simulink model "app_webserver_demo"  (Simulink 7.3)
settings: Solver=FixedStepDiscrete  SolverMode=SingleTasking  StartTime=0.0  StopTime=10.0  RelTol=1e-3
PreLoadFcn:
  | waijung.modelPreload; % Required for working with Waijung Blockset. Do not remove.
undefined symbols (not defined in the file): A0, A1, A2, A3, A7, B0, B1, B10, B11, B12, B13, C1, C2, C3, C4, C5, HSEOSC, LQFP176, STM32F417IG
libraries: waijung_webserver x3, stm32f4_boot_lib x1, simulink x1, stm32f4_io_lib x1, stm32f4_device_config_lib x1
CloseFcn:
  | waijung.modelClose; % Required for working with Waijung Blockset. Do not remove.
settings Model: Creator=Krisada  LastModifiedBy=Krisada
settings OptimizationCC: OptimizeModelRefInitCode=on  LifeSpan=1
settings HardwareCC: ProdEndianess=LittleEndian  ProdHWDeviceType=ARM Compatible->Cortex - M4  TargetEndianess=LittleEndian  TargetHWDeviceType=ARM Compatible->Cortex - M4
settings RTWCC: SystemTargetFile=stm32f4.tlc  GenerateMakefile=off  TemplateMakefile=ert_default_tmf  Description=STM32F4 Target  ProcessScript=stm32f4_make_rtw_hook
settings CodeAppCC: IgnoreCustomStorageClasses=off
settings STFCustomTargetCC: ModelReferenceCompliant=off  CombineOutputUpdateFcns=on  ERTCustomFileBanners=on  SupportContinuousTime=off  SupportNonInlinedSFcns=off  SystemTargetFile=stm32f4.tlc
settings ERTTargetCC: MultiwordLength=2048  ModelReferenceCompliant=off  ParMdlRefBuildCompliant=off  CompOptLevelCompliant=off  ERTFirstTimeCompliant=off  ModelStepFunctionPrototypeControlCompliant=off  CPPClassGenCompliant=off  ExtModeMexFile=noextcomm  InlinedParameterPlacement=NonHierarchical  ERTSrcFileBannerTemplate=stm32f4_code_template.cgt  ERTHdrFileBannerTemplate=stm32f4_code_template.cgt  ERTDataSrcFileTemplate=stm32f4_code_template.cgt  ERTDataHdrFileTemplate=stm32f4_code_template.cgt  ERTCustomFileTemplate=stm32f4_file_process.tlc

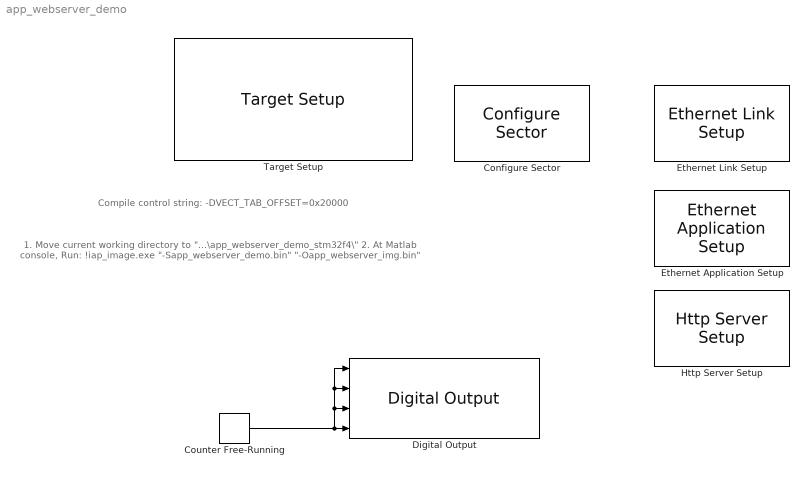
== system app_webserver_demo ==
  note: 1. Move current working directory to "...\app_webserver_demo_stm32f4\"
      | 2. At Matlab console, Run:
      | !iap_image.exe "-Sapp_webserver_demo.bin" "-Oapp_webserver_img.bin"
  note: Compile control string:
      |  -DVECT_TAB_OFFSET=0x20000
  Configure Sector : stm32f4_boot_lib/Configure Sector  conf=Configure  flashorigin=0x8020000  flashlength=0x060000  enableisr=off  usersector=Sector 5: 0x08020000 - 0x0803FFFF  sampletime=-1  sampletimestr=0.001  blockid=ConfigureSector  inputarray=[]  inputlabelarray={}  outputarray=[]  outputlabelarray={}  compat=0  confstr="[\"08020000\",\"5\"]"
  Counter Free-Running : simulink/Sources/Counter Free-Running  SystemSampleTime=-1  NumBits=16  tsamp=0.5
  Digital Output : stm32f4_io_lib/Digital Output  use_bitband=on  port=D  speed=100  porttype=Push Pull  porttypestr=PP  use_pin0=off  use_pin1=off  use_pin2=off  use_pin3=off  use_pin4=off  use_pin5=off  use_pin6=off  use_pin7=off  use_pin8=off  use_pin9=off  use_pin10=off  use_pin11=off  use_pin12=on  use_pin13=on  use_pin14=on  use_pin15=on  pinstr=GPIO_Pin_12 | GPIO_Pin_13 | GPIO_Pin_14 | GPIO_Pin_15  usedpinarray="[0  0  0  0  0  0  0  0  0  0  0  0  1  1  1  1]"  bitbandingstr=|  sampletime=-1  sampletimestr=0.5  blockid=DigitalOutput  enablecustomportlabel=off  globalinit=off  cinputportlabel=In1, In2  coutputportlabel=0
      | #define DigitalOutput_D12 Peripheral_BB(GPIOD->ODR, 12)  /* Output pin */
      | #define DigitalOutput_D13 Peripheral_BB(GPIOD->ODR, 13)  /* Output pin */
      | #define DigitalOutput_D14 Peripheral_BB(GPIOD->ODR, 14)  /* Output pin */
      | #define DigitalOutput_D15 Peripheral_BB(GPIOD->ODR, 15)  /* Output pin */
  Ethernet Application Setup : waijung_webserver/Ethernet Application Setup  conf=Setup  ipaddress=192.168.1.31  netmask=255.255.255.0  gateway=192.168.1.1  macaddress=02-00-00-00-00-00  dhcp=off  timerscaler=10  portpinstr=0  sampletime=0.001  blockid=EthernetApplicationSetup  inputporttype=[]  inputportwidth=[]  inputportlabel={}  outputporttype=[]  outputportwidth=[]  outputportlabel={}  compat=0  optionstring="[\"Dummy\",\"192\",\"168\",\"1\",\"31\",\"255\",\"255\",\"255\",\"0\",\"192\",\"168\",\"1\",\"1\",\"02\",\"00\",\"00\",\"00\",\"00\",\"00\",\"off\",\"10\"]"
  Ethernet Link Setup : waijung_webserver/Ethernet Link Setup  conf=Setup  interfacepin=Profile #1  wj_interfacetype=MII  pin_mdio=A2  pin_mdc=C1  pin_pps=Not used  pin_crs=A0  pin_col=A3  pin_dv=A7  pin_rxclk=A1  pin_rxer=B10  pin_rxd0=C4  pin_rxd1=C5  pin_rxd2=B0  pin_rxd3=B1  pin_txclk=C3  pin_txen=B11  pin_txd0=B12  pin_txd1=B13  pin_txd2=C2  pin_txd3=E2  portpinstr=A0,A1,A2,A3,A7,B0,B1,E2,B10,B11,B12,B13,C1,C2,C3,C4,C5  sampletime=inf  blockid=EthernetLinkSetup  inputporttype=[]  inputportwidth=[]  inputportlabel={}  outputporttype=[]  outputportwidth=[]  outputportlabel={}  compat=0  optionstring="[\"xxx\",\"on\",\"on\",\"on\",\"off\",\"on\",\"off\",\"off\",\"off\",\"off\",\"on\",\"on\",\"on\",\"on\",\"on\",\"on\",\"on\",\"off\",\"on\",\"on\",\"on\",\"on\",\"on\",\"on\",\"on\",\"on\",\"on\",\"on\",\"A\",\"0\",\"A\",\"1\",\"A\",\"2\",\"A\",\"3\",\"A\",\"7\",\"B\",\"0\",\"B\",\"1\",\"N\",\"ot used\",\"E\",\"2\",\"B\",\"10\",\"B\",\"11\",\"B\",\"12\",\"B\",\"13\",\"C\",\"1\",\"C\",\"2\",\"C\",\"3\",\"C\",\"4\",\"C\",\"5\",\"MII\"]"
  Http Server Setup : waijung_webserver/Http Server Setup  conf=Setup  port=80  ssl=Disable  sqlite=Disable  iap=Disable  mempool=8  debugport=Disable  portpinstr=0  sampletime=inf  blockid=HttpServerSetup  inputporttype=[]  inputportwidth=[]  inputportlabel={}  outputporttype=[]  outputportwidth=[]  outputportlabel={}  compat=0  optionstring="[\"80\",\"0\",\"0\",\"Disable\",\"Disable\",\"8\",\"14.03a\",\"\",\"\",\"\"]"
  Target Setup : stm32f4_device_config_lib/Target Setup  Priority=100  compiler=GNU ARM  previous_compiler=GNU ARM  mcu=STM32F417IG (LQFP176)  mcustr=STM32F417IG  clockconfig=HSEOSC-8MHz  system_stm32f4xx_c_path=F:\trunk\targets\stm32f4_target\stm32f4\utils\system_stm32f4xx_default\STM32F40_41xxx\hseosc8mhz  showmemoryconfiguration=off  stacksize=0x2000  heapsize=0x2000  enableautocompiledownload=on  fullchiperase=off  programmerinterface=None  editctrlstr=on  compilercontrolstr=$(patsubst %, -I%, .) -mcpu=cortex-m4 -mthumb -mthumb-interwork -mfloat-abi=hard -mfpu=fpv4-sp-d16 -ffast-math -Wall -Wextra -Ofast  assemblercontrolstr=$(patsubst %, -I%, .) -mcpu=cortex-m4 -mthumb -mthumb-interwork -mfloat-abi=hard -mfpu=fpv4-sp-d16 -ffast-math -Wall -Wextra -Ofast -Wa,-amhls=$(<:.s=.lst) -D__STACK_SIZE=$(STACK_SIZE) -D__HEAP_SIZE=$(HEAP_SIZE)  linkercontrolstr=-T$(LD_SCRIPT) -g -Wl,-Map=$(MAP),--cref,--no-warn-mismatch -mcpu=cortex-m4 -mthumb -mthumb-interwork -mfloat-abi=hard -mfpu=fpv4-sp-d16 -specs=nosys.specs  runafterdownload=on  execprofile=None  profileruart=3  profilerbaud=500000  profilertxpin=D8  profilerinitstr=0.001,168000000,168000,500000,0  manualsetsampletime=off  sampletime=0.001  blockid=TargetSetup  systickreloadvalue=168000  hseval=8000000  lastprofileruart=3  hclk=168000000  flashorigin=0x8020000  flashlength=0x060000  ramorigin=0x20000000  ramlength=128k  useextram=off
  wires:
  Counter Free-Running/1 -> Digital Output/4, Digital Output/3, Digital Output/2, Digital Output/1
